simulink subsystem "Measurement_sim"  (R2024a)
settings: Solver=VariableStepAuto  StartTime=0.0  StopTime=10.0  RelTol=1e-3
undefined symbols (not defined in the file or in its folder): NoiseCov, Orbit_Incl
settings Model: Creator=ruimi  LastModifiedBy=ruimi

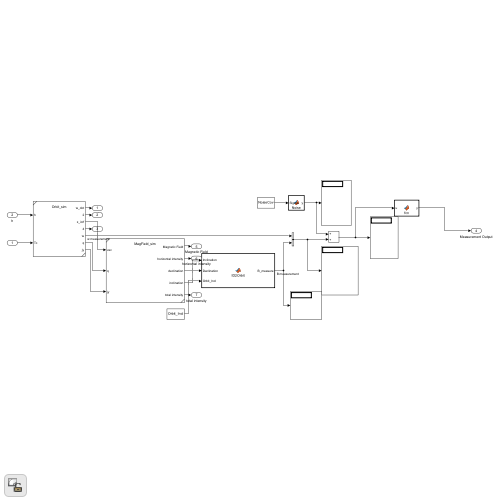
[thumbnail: Simulink's stored preview of the top-level diagram]
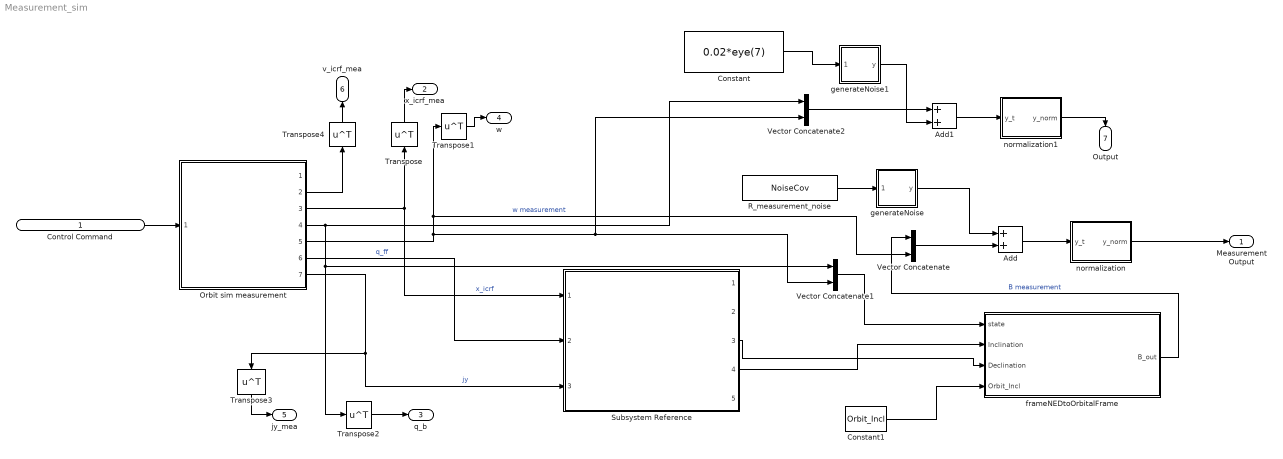
== system Measurement_sim ==
  Control Command : Inport
  Add : Sum  Priority=7
  Add1 : Sum
  Constant : Constant  Value=0.02*eye(7)
  Constant1 : Constant  Value=Orbit_Incl
  Orbit sim measurement : Subsystem  Priority=2  ReferencedSubsystem=Orbit_sim_measurement
  R_measurement_noise : Constant  Value=NoiseCov
  Subsystem Reference : Subsystem  Priority=3  ReferencedSubsystem=MagField_mea_sim
  Transpose{,1..4} (5 alike) : Math  Priority=3  Operator=transpose
  Vector Concatenate : Concatenate  Priority=5
  Vector Concatenate1 : Concatenate  Priority=5
  Vector Concatenate2 : Concatenate
  frameNEDtoOrbitalFrame : MATLAB Function  Priority=4  TreatAsAtomicUnit=on
  generateNoise : MATLAB Function  Priority=1  TreatAsAtomicUnit=on
  generateNoise1 : MATLAB Function  Priority=1  TreatAsAtomicUnit=on
  normalization : MATLAB Function  TreatAsAtomicUnit=on
  normalization1 : MATLAB Function  TreatAsAtomicUnit=on
  Measurement Output : Outport
  x_icrf_mea : Outport  Port=2
  q_b : Outport  Port=3
  w : Outport  Port=4
  jy_mea : Outport  Port=5
  v_icrf_mea : Outport  Port=6
  Output : Outport  Port=7
  wires:
  Add/1 -> normalization/1(y_t)
  Orbit sim measurement/3 -> Transpose/1, Subsystem Reference/1  "x_icrf"
  Control Command/1 -> Orbit sim measurement/1
  Orbit sim measurement/7 -> Transpose3/1, Subsystem Reference/3  "jy"
  Vector Concatenate/1 -> Add/2
  generateNoise/1(y) -> Add/1
  Orbit sim measurement/5 -> Vector Concatenate1/2, Vector Concatenate2/2, Vector Concatenate/2, Transpose1/1  "w measurement"
  R_measurement_noise/1 -> generateNoise/1(Sigma)
  Orbit sim measurement/4 -> Vector Concatenate2/1, Transpose2/1, Vector Concatenate1/1
  Transpose/1 -> x_icrf_mea/1
  Transpose1/1 -> w/1
  Transpose2/1 -> q_b/1
  Transpose3/1 -> jy_mea/1
  Orbit sim measurement/2 -> Transpose4/1
  Transpose4/1 -> v_icrf_mea/1
  normalization/1(y_norm) -> Measurement Output/1
  Orbit sim measurement/6 -> Subsystem Reference/2  "q_ff"
  Constant1/1 -> frameNEDtoOrbitalFrame/4(Orbit_Incl)
  Subsystem Reference/4 -> frameNEDtoOrbitalFrame/2(Inclination)
  Subsystem Reference/3 -> frameNEDtoOrbitalFrame/3(Declination)
  Vector Concatenate1/1 -> frameNEDtoOrbitalFrame/1(state)
  frameNEDtoOrbitalFrame/1(B_out) -> Vector Concatenate/1  "B measurement"
  Vector Concatenate2/1 -> Add1/1
  generateNoise1/1(y) -> Add1/2
  Constant/1 -> generateNoise1/1(Sigma)
  Add1/1 -> normalization1/1(y_t)
  normalization1/1(y_norm) -> Output/1

== matlab function Measurement_sim/generateNoise ==
  data: y output; Sigma input
function y = Noise(Sigma)
secs = mod(mod(now,1)*1000000, 1000);
rng(secs);
mu = [0 0 0 0 0 0] ; %mean is zero for noise
%covariance is constant throughout, we take the input
y_temp = mvnrnd(mu,Sigma,1);
y = transpose(y_temp);
%disp(y)
end

== matlab function Measurement_sim/normalization ==
  data: y_t input; y_norm output
function y_norm = normalizeY(y_t)
y_norm = zeros(6,1);
y_norm(1:3) = y_t(1:3)/norm(y_t(1:3));
y_norm(4:6) = y_t(4:6);

== matlab function Measurement_sim/frameNEDtoOrbitalFrame ==
  data: state input; Inclination input; B_out output; Declination input; Orbit_Incl input
function B_out= ID2Orbit(state, Inclination,Declination, Orbit_Incl)
%disp('enter NED in measurement')
[Down_dir,Omega_dir,Other_dir] = MagID2Orbit(Inclination,Declination, Orbit_Incl);
B_measure = [Down_dir;Omega_dir;Other_dir]/norm([Down_dir,Omega_dir,Other_dir]);
B = h_t(state,B_measure);
B_out = B(1:3);
end

== matlab function Measurement_sim/generateNoise1 ==
  data: y output; Sigma input
function y = Noise(Sigma)
secs = mod(mod(now,1)*1000000, 1000);
rng(secs);
mu = [0 0 0 0 0 0 0] ; %mean is zero for noise
%covariance is constant throughout, we take the input
y_temp = mvnrnd(mu,Sigma,1);
y = transpose(y_temp);
end

== matlab function Measurement_sim/normalization1 ==
  data: y_t input; y_norm output
function y_norm = normalizeY(y_t)
y_norm = zeros(7,1);
y_norm(1:4) = y_t(1:4)/norm(y_t(1:4));
y_norm(5:7) = y_t(5:7);
